simulink model "project5_week1"  (R2020b)
settings: Solver=VariableStepAuto  StartTime=0.0  StopTime=10.0  RelTol=1e-3
undefined symbols (not defined in the file): C, R
settings Model: Creator=RASIKA MALGI  LastModifiedBy=RASIKA MALGI

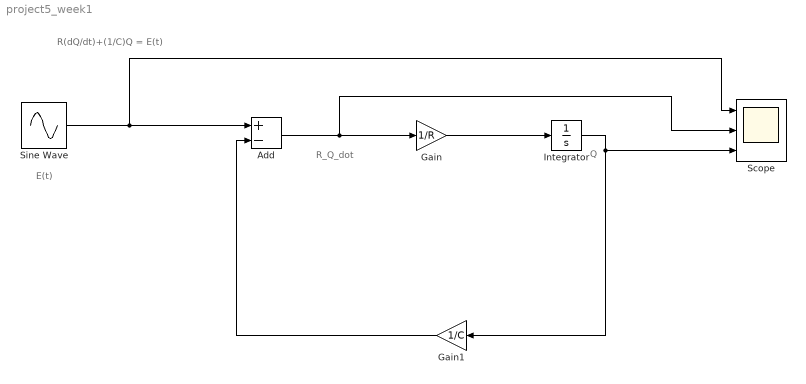
== system project5_week1 ==
  note: R(dQ/dt)+(1/C)Q = E(t)
  note: Q
  note: R_Q_dot
  note: E(t)
  Add : Sum  Inputs=+-
  Gain : Gain  Gain=1/R
  Gain1 : Gain  Gain=1/C
  Integrator : Integrator  InitialCondition=4
  Scope : Scope  NumInputPorts=3
  Sine Wave : Sin  SampleTime=0
  wires:
  Sine Wave/1 -> Scope/1, Add/1
  Add/1 -> Scope/2, Gain/1
  Gain/1 -> Integrator/1
  Integrator/1 -> Gain1/1, Scope/3
  Gain1/1 -> Add/2
